simulink model "TST_BusSelectorProblem"  (Simulink 7.4)
settings: Solver=FixedStepDiscrete  StartTime=0.0  StopTime=10.0  FixedStep=0.02  RelTol=1e-3
settings Model: Creator=kharthforeign  LastModifiedBy=kharthforeign  BufferReuse=off
settings DataIOCC: SaveOutput=off  SignalLogging=off  SaveTime=off
settings OptimizationCC: BlockReduction=off  ConditionallyExecuteInputs=off  OptimizeBlockIOStorage=off  BufferReuse=off  ExpressionFolding=off  LocalBlockOutputs=off  InitFltsAndDblsToZero=on

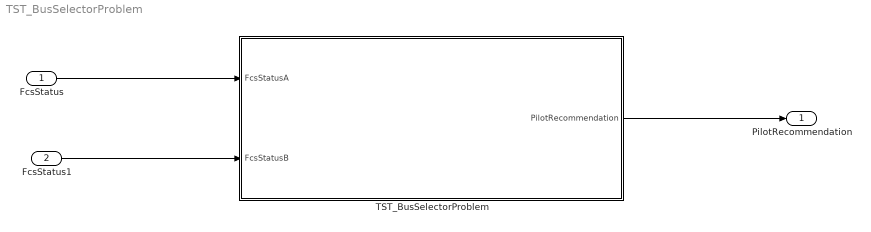
== system TST_BusSelectorProblem ==
  FcsStatus : Inport  UseBusObject=on  OutDataType=fixdt(1, 16)  OutScaling=2^0
      settings: BusObject=FCS_FlightControlSystem_Status
  FcsStatus1 : Inport  Port=2  UseBusObject=on  OutDataType=fixdt(1, 16)  OutScaling=2^0
      settings: BusObject=FCS_FlightControlSystem_Status
  TST_BusSelectorProblem : Subsystem  TreatAsAtomicUnit=on
  PilotRecommendation : Outport  PortDimensions=1  DataType=uint32  OutDataType=Enum: GBL_Definitions_EjectionCmd  OutDataTypeStr=uint32
  wires:
  FcsStatus/1 -> TST_BusSelectorProblem/1(FcsStatusA)
  TST_BusSelectorProblem/1(PilotRecommendation) -> PilotRecommendation/1
  FcsStatus1/1 -> TST_BusSelectorProblem/2(FcsStatusB)

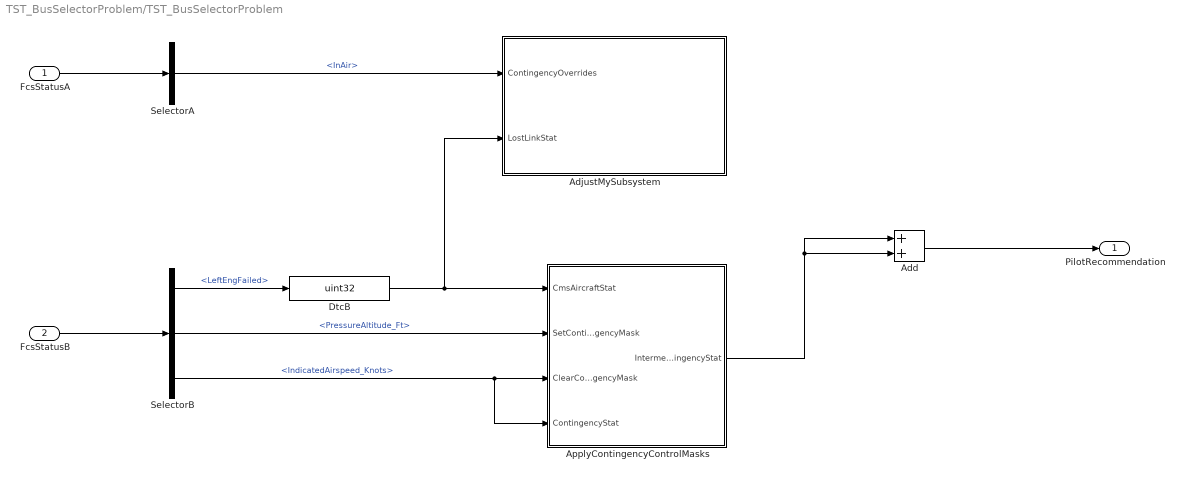
== system TST_BusSelectorProblem/TST_BusSelectorProblem ==
  FcsStatusA : Inport  UseBusObject=on  OutDataType=fixdt(1, 16)  OutScaling=2^0
      settings: BusObject=FCS_FlightControlSystem_Status
  FcsStatusB : Inport  Port=2  UseBusObject=on  OutDataType=fixdt(1, 16)  OutScaling=2^0
      settings: BusObject=FCS_FlightControlSystem_Status
  Add : Sum  OutDataType=fixdt(1, 16)  OutScaling=2^-10
  AdjustMySubsystem : Subsystem  TreatAsAtomicUnit=on
  ApplyContingencyControlMasks : Subsystem  TreatAsAtomicUnit=on
  DtcB : DataTypeConversion  OutDataTypeMode=uint32  OutDataType=fixdt(1, 16)  OutScaling=2^0  OutDataTypeStr=uint32
  SelectorA : BusSelector  OutputSignals=InAir
  SelectorB : BusSelector  OutputSignals=LeftEngFailed,PressureAltitude_Ft,IndicatedAirspeed_Knots
  PilotRecommendation : Outport  PortDimensions=1  DataType=uint32  OutDataType=Enum: GBL_Definitions_EjectionCmd  OutDataTypeStr=uint32
  wires:
  FcsStatusA/1 -> SelectorA/1
  FcsStatusB/1 -> SelectorB/1
  SelectorA/1 -> AdjustMySubsystem/1(ContingencyOverrides)  "<InAir>"
  SelectorB/1 -> DtcB/1  "<LeftEngFailed>"
  DtcB/1 -> AdjustMySubsystem/2(LostLinkStat), ApplyContingencyControlMasks/1(CmsAircraftStat)
  SelectorB/2 -> ApplyContingencyControlMasks/2(SetContingencyMask)  "<PressureAltitude_Ft>"
  SelectorB/3 -> ApplyContingencyControlMasks/3(ClearContingencyMask), ApplyContingencyControlMasks/4(ContingencyStat)  "<IndicatedAirspeed_Knots>"
  Add/1 -> PilotRecommendation/1
  ApplyContingencyControlMasks/1(IntermediateContingencyStat) -> Add/2, Add/1

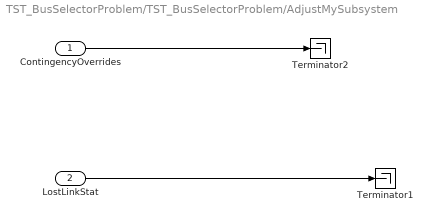
== system TST_BusSelectorProblem/TST_BusSelectorProblem/AdjustMySubsystem ==
  ContingencyOverrides : Inport  OutDataType=fixdt(1, 16)  OutScaling=2^0
  LostLinkStat : Inport  Port=2  OutDataType=fixdt(1, 16)  OutScaling=2^0
  Terminator1 : Terminator
  Terminator2 : Terminator
  wires:
  ContingencyOverrides/1 -> Terminator2/1
  LostLinkStat/1 -> Terminator1/1

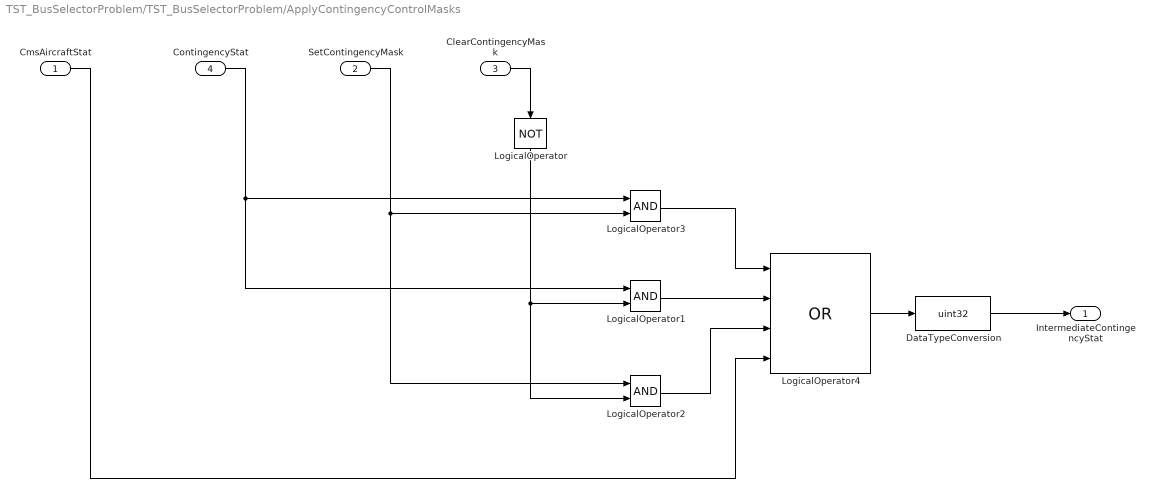
== system TST_BusSelectorProblem/TST_BusSelectorProblem/ApplyContingencyControlMasks ==
  CmsAircraftStat : Inport  OutDataType=fixdt(1, 16)  OutScaling=2^0
  SetContingencyMask : Inport  Port=2  OutDataType=fixdt(1, 16)  OutScaling=2^0
  ClearContingencyMask : Inport  Port=3  OutDataType=fixdt(1, 16)  OutScaling=2^0
  ContingencyStat : Inport  Port=4  OutDataType=fixdt(1, 16)  OutScaling=2^0
  DataTypeConversion : DataTypeConversion  OutDataTypeMode=uint32  OutDataType=fixdt(1, 16)  OutScaling=2^0  OutDataTypeStr=uint32
  LogicalOperator : Logic  Operator=NOT  AllPortsSameDT=off  OutDataTypeMode=boolean  LogicDataType=fixdt(0, 8)  OutDataTypeStr=boolean
  LogicalOperator1 : Logic  AllPortsSameDT=off  OutDataTypeMode=boolean  LogicDataType=fixdt(0, 8)  OutDataTypeStr=boolean
  LogicalOperator2 : Logic  AllPortsSameDT=off  OutDataTypeMode=boolean  LogicDataType=fixdt(0, 8)  OutDataTypeStr=boolean
  LogicalOperator3 : Logic  AllPortsSameDT=off  OutDataTypeMode=boolean  LogicDataType=fixdt(0, 8)  OutDataTypeStr=boolean
  LogicalOperator4 : Logic  Operator=OR  Inputs=4  AllPortsSameDT=off  OutDataTypeMode=boolean  LogicDataType=fixdt(0, 8)  OutDataTypeStr=boolean
  IntermediateContingencyStat : Outport  OutDataType=fixdt(1, 16)  OutScaling=2^0
  wires:
  LogicalOperator3/1 -> LogicalOperator4/1
  LogicalOperator1/1 -> LogicalOperator4/2
  LogicalOperator2/1 -> LogicalOperator4/3
  ClearContingencyMask/1 -> LogicalOperator/1
  SetContingencyMask/1 -> LogicalOperator2/1, LogicalOperator3/2
  LogicalOperator/1 -> LogicalOperator2/2, LogicalOperator1/2
  ContingencyStat/1 -> LogicalOperator1/1, LogicalOperator3/1
  CmsAircraftStat/1 -> LogicalOperator4/4
  LogicalOperator4/1 -> DataTypeConversion/1
  DataTypeConversion/1 -> IntermediateContingencyStat/1
